simulink model "sim_mpc"  (R2020a)
settings: Solver=ode1  StartTime=0.0  StopTime=sim_time  FixedStep=0.00025  RelTol=1e-3
undefined symbols (not defined in the file): accl, accl_param, accl_param_limit, accl_param_n, alpha, base_alpha, base_time, counter, decel, dist, ego_accl, ego_alpha, ego_dist, ego_state, ego_v, ego_w, end_v, end_w, k_theta, k_x, k_y, kanayama_gain, limit_accl_ratio_cnt, limit_decel_ratio_cnt, limit_time_count, param_alpha, pow_n, sla, sla_param, slip_gain, state, test_mode, tgt_angle, tgt_dist, v, v_max, w, w_max
settings Model: Creator=nao12  LastModifiedBy=nao12
settings DataIOCC: SaveOutput=off  SignalLogging=off  DSMLogging=off  SaveTime=off  ReturnWorkspaceOutputs=off
settings OptimizationCC: DefaultParameterBehavior=Inlined  EnhancedBackFolding=on  PassReuseOutputArgsAs=Individual arguments  OptimizeBlockOrder=speed  DifferentSizesBufferReuse=on  OptimizationCustomize=off  EfficientTunableParamExpr=on
settings DebuggingCC: ParameterTunabilityLossMsg=error  ArithmeticOperatorsInVariantConditions=warning
settings HardwareCC: ProdBitPerPointer=32  ProdBitPerSizeT=32  ProdBitPerPtrDiffT=32  ProdLargestAtomicFloat=None  ProdWordSize=32  ProdHWDeviceType=Renesas->RX
settings ModelReferenceCC: UpdateModelReferenceTargets=IfOutOfDate
settings SFSimCC: SimCustomHeaderCode="#include \"bus.h\""  SimUserIncludeDirs=../include/  MATLABDynamicMemAlloc=off  CustomCodeUndefinedFunction=UseInterfaceOnly
settings RTWCC: SystemTargetFile=ert.tlc  GenCodeOnly=on  TemplateMakefile=ert_default_tmf  GenerateReport=on  RTWUseSimCustomCode=on  CustomHeaderCode="#include \"bus.h\""  CustomInclude=../include/  IncludeHyperlinkInReport=on  LaunchReport=on  GenerateTraceInfo=on  GenerateTraceReport=on  GenerateTraceReportSl=on  GenerateTraceReportSf=on  GenerateTraceReportEml=on
settings CodeAppCC: ForceParamTrailComments=on  IgnoreCustomStorageClasses=off  OperatorAnnotations=on  SimulinkDataObjDesc=on  SFDataObjDesc=on  InsertBlockDesc=on
settings ERTTargetCC: TargetLangStandard=C99 (ISO)  GenerateSampleERTMain=on  SupportAbsoluteTime=off  MultiInstanceERTCode=on  CodeInterfacePackaging=Reusable function  SupportComplex=off  InlinedParameterPlacement=NonHierarchical  ERTCustomFileTemplate=example_file_process.tlc  EnableUserReplacementTypes=on

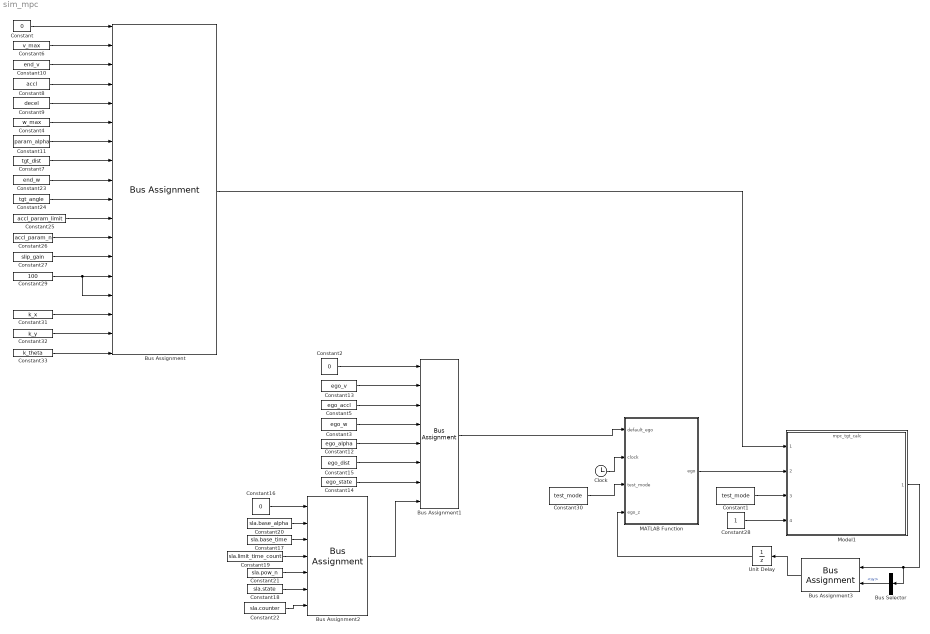
== system sim_mpc ==
  Bus Assignment : BusAssignment  AssignedSignals=v_max,end_v,accl,decel,w_max,alpha,tgt_dist,end_w,tgt_angle,accl_param.limit,accl_param.n,slip_gain,limit_accl_ratio_cnt,limit_decel_ratio_cnt,kanayama_gain.k_x,kanayama_gain.k_y,kanayama_gain.k_theta
  Bus Assignment1 : BusAssignment  AssignedSignals=v,accl,w,alpha,dist,state,sla_param
  Bus Assignment2 : BusAssignment  AssignedSignals=base_alpha,base_time,limit_time_count,pow_n,state,counter
  Bus Assignment3 : BusAssignment  AssignedSignals=slip_point.w
  Bus Selector : BusSelector  OutputSignals=w
  Clock : Clock
  Constant : Constant  Value=0  OutDataTypeStr=Bus: t_tgt
  Constant1 : Constant  Value=test_mode  OutDataTypeStr=int32
  Constant10 : Constant  Value=end_v  OutDataTypeStr=single
  Constant11 : Constant  Value=param_alpha  OutDataTypeStr=single
  Constant12 : Constant  Value=ego_alpha  OutDataTypeStr=single
  Constant13 : Constant  Value=ego_v  OutDataTypeStr=single
  Constant14 : Constant  Value=ego_state
  Constant15 : Constant  Value=ego_dist  OutDataTypeStr=single
  Constant16 : Constant  Value=0  OutDataTypeStr=Bus: t_slalom
  Constant17 : Constant  Value=sla.base_time  OutDataTypeStr=single
  Constant18 : Constant  Value=sla.state  OutDataTypeStr=int8
  Constant19 : Constant  Value=sla.limit_time_count  OutDataTypeStr=single
  Constant2 : Constant  Value=0  OutDataTypeStr=Bus: t_ego
  Constant20 : Constant  Value=sla.base_alpha  OutDataTypeStr=single
  Constant21 : Constant  Value=sla.pow_n  OutDataTypeStr=single
  Constant22 : Constant  Value=sla.counter  OutDataTypeStr=int32
  Constant23 : Constant  Value=end_w  OutDataTypeStr=single
  Constant24 : Constant  Value=tgt_angle  OutDataTypeStr=single
  Constant25 : Constant  Value=accl_param_limit  OutDataTypeStr=single
  Constant26 : Constant  Value=accl_param_n  OutDataTypeStr=single
  Constant27 : Constant  Value=slip_gain  OutDataTypeStr=single
  Constant28 : Constant  OutDataTypeStr=int32
  Constant29 : Constant  Value=100  OutDataTypeStr=single
  Constant3 : Constant  Value=ego_w  OutDataTypeStr=single
  Constant30 : Constant  Value=test_mode  OutDataTypeStr=int32
  Constant31 : Constant  Value=k_x  OutDataTypeStr=single
  Constant32 : Constant  Value=k_y  OutDataTypeStr=single
  Constant33 : Constant  Value=k_theta  OutDataTypeStr=single
  Constant4 : Constant  Value=w_max  OutDataTypeStr=single
  Constant5 : Constant  Value=ego_accl  OutDataTypeStr=single
  Constant6 : Constant  Value=v_max  OutDataTypeStr=single
  Constant7 : Constant  Value=tgt_dist  OutDataTypeStr=single
  Constant8 : Constant  Value=accl  OutDataTypeStr=single
  Constant9 : Constant  Value=decel  OutDataTypeStr=single
  MATLAB Function : MATLAB Function  TreatAsAtomicUnit=on
  Model1 : ModelReference  ModelNameDialog=mpc_tgt_calc.slx  SimulationMode=Normal  ModelReferenceVersion=1.341
  Unit Delay : UnitDelay  SampleTime=-1  HasFrameUpgradeWarning=on
  wires:
  Model1/1 -> Bus Selector/1, Bus Assignment3/1
  Constant/1 -> Bus Assignment/1
  Bus Assignment/1 -> Model1/1
  Constant1/1 -> Model1/3
  Constant2/1 -> Bus Assignment1/1
  Bus Assignment1/1 -> MATLAB Function/1(default_ego)
  MATLAB Function/1(ego) -> Model1/2
  Constant6/1 -> Bus Assignment/2
  Constant8/1 -> Bus Assignment/4
  Constant9/1 -> Bus Assignment/5
  Constant4/1 -> Bus Assignment/6
  Constant11/1 -> Bus Assignment/7
  Constant7/1 -> Bus Assignment/8
  Constant10/1 -> Bus Assignment/3
  Constant13/1 -> Bus Assignment1/2
  Constant3/1 -> Bus Assignment1/4
  Constant5/1 -> Bus Assignment1/3
  Constant12/1 -> Bus Assignment1/5
  Constant15/1 -> Bus Assignment1/6
  Constant14/1 -> Bus Assignment1/7
  Constant16/1 -> Bus Assignment2/1
  Bus Assignment2/1 -> Bus Assignment1/8
  Constant20/1 -> Bus Assignment2/2
  Constant17/1 -> Bus Assignment2/3
  Constant19/1 -> Bus Assignment2/4
  Constant18/1 -> Bus Assignment2/6
  Constant21/1 -> Bus Assignment2/5
  Constant22/1 -> Bus Assignment2/7
  Constant23/1 -> Bus Assignment/9
  Constant24/1 -> Bus Assignment/10
  Clock/1 -> MATLAB Function/2(clock)
  Unit Delay/1 -> MATLAB Function/4(ego_z)
  Constant25/1 -> Bus Assignment/11
  Constant26/1 -> Bus Assignment/12
  Constant27/1 -> Bus Assignment/13
  Constant28/1 -> Model1/4
  Bus Assignment3/1 -> Unit Delay/1
  Bus Selector/1 -> Bus Assignment3/2  "<w>"
  Constant29/1 -> Bus Assignment/15, Bus Assignment/14
  Constant30/1 -> MATLAB Function/3(test_mode)
  Constant31/1 -> Bus Assignment/16
  Constant32/1 -> Bus Assignment/17
  Constant33/1 -> Bus Assignment/18

== matlab function sim_mpc/MATLAB Function ==
  data: default_ego input; ego output Bus: t_ego; clock input; test_mode input; ego_z input; sim_time parameter
function ego  = fcn( default_ego, clock, test_mode, ego_z, sim_time)
   ego = debug( default_ego, clock, ego_z, test_mode, sim_time);
end
